simulink model "GeneratorRectifierModel"  (R2021a)
settings: Solver=FixedStepAuto  StartTime=0.0  StopTime=t  FixedStep=tstep  RelTol=1e-3
values from neighbouring files (symbols this model uses):
  gen_catastrophic_fault_toggle = input('   0 = no fault  -or-  1 = fault: ')    [Run_GeneratorRectifierBoostConverterInverterMotorModel.m]    (also in Run_GeneratorRectifierBoostConverterModel.m; Run_GeneratorRectifierBuckConverterModel.m; Run_GeneratorRectifierModel.m)
  rect_catastrophic_fault_toggle = input('   0 = no fault  -or-  1 = fault: ')    [Run_GeneratorRectifierBoostConverterInverterMotorModel.m]    (also in Run_GeneratorRectifierBoostConverterModel.m; Run_GeneratorRectifierBuckConverterModel.m; Run_GeneratorRectifierModel.m)
libraries: PB_Library_Master_Working x2
settings Model: Creator=sfaulk  LastModifiedBy=sfaulk

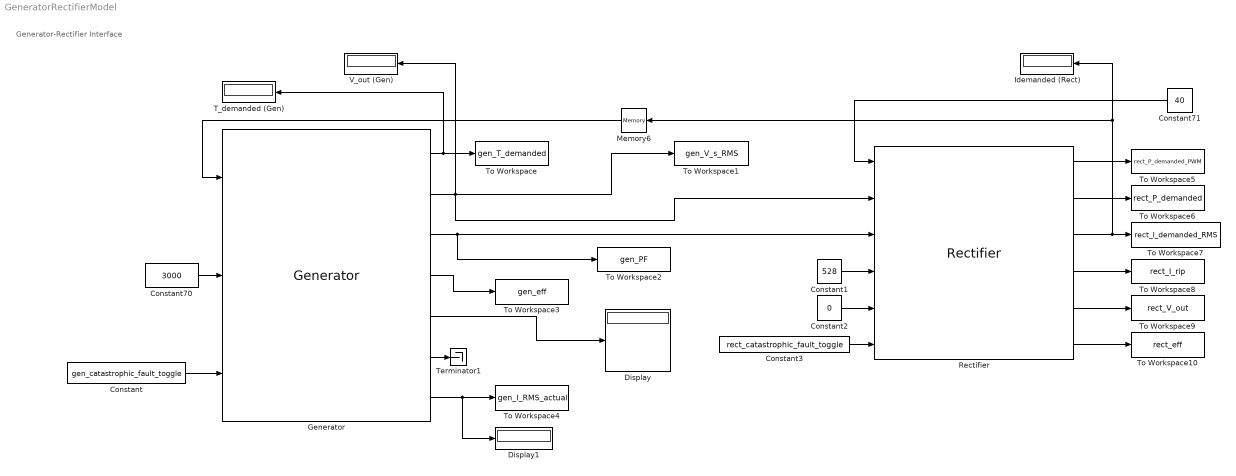
== system GeneratorRectifierModel ==
  note: Generator-Rectifier Interface
  Constant : Constant  Value=gen_catastrophic_fault_toggle
  Constant1 : Constant  Value=528
  Constant2 : Constant  Value=0
  Constant3 : Constant  Value=rect_catastrophic_fault_toggle
  Constant70 : Constant  Value=3000
  Constant71 : Constant  Value=40
  Display : Display
  Display1 : Display
  Generator : PB_Library_Master_Working/Generator  pp=3  flux_m=0.8  R_s=0.6  L_s=0.02  P_Fe_Nom=900  S_nom=3000  T_nom=70  P_out_max=30000000  I_max=50  P_in_max=30000  T_max=80  MassEst_M=-1080970  Poles_i=6  R_s_i=.032  L_s_i=.00086+0.00029  S_nom_i=4000  T_nom_i=70  P_out_max_i=22000  I_max_i=36.5  P_in_max_i=30000  K_i=121  V_nom_i=368  T_max_i=80  CalculatePFe=Compute iron losses automatically  P_Fe_Nom_i=0  I_nom_i=36.5  PF_nom_i=0.99  P_Fe_Calc_Flag=1
      link override Constant2: Value=0.1
      link override Copper Losses/Constant: Value=0.01
      link override Copper Losses/Constant1: Value=0.01
      link override Copper Losses/Degradation Parameter Multiplier/From14: GotoTag=genDI
      link override Copper Losses/Degradation Parameter Multiplier/From15: GotoTag=genDF
      link override Copper Losses/Degradation Parameter Multiplier1/From14: GotoTag=genDI
      link override Copper Losses/Degradation Parameter Multiplier1/From15: GotoTag=genDF
      link override Copper Losses/From1: GotoTag=DM
      link override Copper Losses/From16: GotoTag=DM
      link override Degradation Input Block/Aging Input: Value=degradation_input
      link override Degradation Input Block/Degradation Input Value: Value=gen_degradation_input
      link override Degradation Input Block/Goto: GotoTag=DI  TagVisibility=global
      link override Degradation Parameter Multiplier/From14: GotoTag=genDI
      link override Degradation Parameter Multiplier/From15: GotoTag=genDF
      link override Field Weakening and d current /Constant2: Value=0.1
      link override Field Weakening and d current /Constant3: Value=0.1
      link override Field Weakening and d current /Degradation Parameter Multiplier/From14: GotoTag=genDI
      link override Field Weakening and d current /Degradation Parameter Multiplier/From15: GotoTag=genDF
      link override Field Weakening and d current /Switch: Threshold=S_nom
      link override Goto4: GotoTag=genDF  TagVisibility=global
      link override Goto6: GotoTag=genDI  TagVisibility=global
      link override Iron Loss/Constant1: Value=0.01
      link override Iron Loss/Constant2: Value=0.1
      link override Iron Loss/Degradation Parameter Multiplier/From14: GotoTag=genDI
      link override Iron Loss/Degradation Parameter Multiplier/From15: GotoTag=genDF
      link override Vdq/Constant: Value=0.01
      link override Vdq/Constant1: Value=0.1
      link override Vdq/Constant2: Value=0.01
      link override Vdq/Degradation Parameter Multiplier/From14: GotoTag=genDI
      link override Vdq/Degradation Parameter Multiplier/From15: GotoTag=genDF
      link override Vdq/Degradation Parameter Multiplier1/From14: GotoTag=genDI
      link override Vdq/Degradation Parameter Multiplier1/From15: GotoTag=genDF
      link override Vdq/Degradation Parameter Multiplier2/From14: GotoTag=genDI
      link override Vdq/Degradation Parameter Multiplier2/From15: GotoTag=genDF
  Idemanded (Rect) : Display
  Memory6 : Memory
  Rectifier : PB_Library_Master_Working/Rectifier  T_M=[25 175]  u_D_M=[1.16666666666667 0.999999999999998]  u_ce0_M=[0.971428571428571 0.848275862068965]  R_c_M=[0.0285714285714286 0.0551724137931034]  R_D_M=[0.0238095238095238 0.0294117647058824]  E0_M=[6.00000000000002e-05 6.00000000000002e-05]  E1_M=[5.6e-05 5.6e-05]  f_sw_M=30000  L_s_M=0.1  P_max_I=22000  V_phase_I=600  f_sw_I=0  L_s_I=0.1
      link override Degradation Input Block/Degradation Input Value: Value=rect_degradation_input
      link override Diode Conduction Losses1/1-D Lookup Table u_D0: Table=u_D_M
      link override Goto1: GotoTag=rectDF  TagVisibility=global
      link override Goto2: GotoTag=rectDI  TagVisibility=global
      link override IGBT Switching Losses1/1-D Lookup Table E1: Table=E1_M/rect_ans.E1_M_aDF.Data(end)
      link override IGBT Switching Losses1/Constant1: Value=rect_ans.f_sw_M_aDF.Data(end)
      link override IGBT Switching Losses1/Degradation Parameter Multiplier/From14: GotoTag=rectDI
      link override IGBT Switching Losses1/Degradation Parameter Multiplier/From15: GotoTag=rectDF
      link override I_Ripple1/Constant1: Value=-0.1
      link override I_Ripple1/Degradation Parameter Multiplier/From14: GotoTag=rectDI
      link override I_Ripple1/Degradation Parameter Multiplier/From15: GotoTag=rectDF
  T_demanded (Gen) : Display
  Terminator1 : Terminator
  To Workspace : ToWorkspace  VariableName=gen_T_demanded  SaveFormat=Timeseries  SampleTime=-1
  To Workspace1 : ToWorkspace  VariableName=gen_V_s_RMS  SaveFormat=Timeseries  SampleTime=-1
  To Workspace10 : ToWorkspace  VariableName=rect_eff  SaveFormat=Timeseries  SampleTime=-1
  To Workspace2 : ToWorkspace  VariableName=gen_PF  SaveFormat=Timeseries  SampleTime=-1
  To Workspace3 : ToWorkspace  VariableName=gen_eff  SaveFormat=Timeseries  SampleTime=-1
  To Workspace4 : ToWorkspace  VariableName=gen_I_RMS_actual  SaveFormat=Timeseries  SampleTime=-1
  To Workspace5 : ToWorkspace  VariableName=rect_P_demanded_PWM  SaveFormat=Timeseries  SampleTime=-1
  To Workspace6 : ToWorkspace  VariableName=rect_P_demanded  SaveFormat=Timeseries  SampleTime=-1
  To Workspace7 : ToWorkspace  VariableName=rect_I_demanded_RMS  SaveFormat=Timeseries  SampleTime=-1
  To Workspace8 : ToWorkspace  VariableName=rect_I_rip  SaveFormat=Timeseries  SampleTime=-1
  To Workspace9 : ToWorkspace  VariableName=rect_V_out  SaveFormat=Timeseries  SampleTime=-1
  V_out (Gen) : Display
  wires:
  Constant/1 -> Generator/3
  Constant71/1 -> Rectifier/1
  Rectifier/3 -> To Workspace7/1, Memory6/1, Idemanded (Rect)/1
  Memory6/1 -> Generator/1
  Constant70/1 -> Generator/2
  Generator/7 -> Display1/1, To Workspace4/1
  Generator/3 -> To Workspace2/1, Rectifier/3
  Generator/1 -> To Workspace/1, T_demanded (Gen)/1
  Generator/4 -> To Workspace3/1
  Generator/5 -> Display/1
  Generator/6 -> Terminator1/1
  Generator/2 -> V_out (Gen)/1, Rectifier/2, To Workspace1/1
  Constant1/1 -> Rectifier/4
  Constant2/1 -> Rectifier/5
  Constant3/1 -> Rectifier/6
  Rectifier/1 -> To Workspace5/1
  Rectifier/2 -> To Workspace6/1
  Rectifier/4 -> To Workspace8/1
  Rectifier/5 -> To Workspace9/1
  Rectifier/6 -> To Workspace10/1
